simulink model "ConImpMulti2Robo_v1"  (R2015b)
settings: Solver=ode1  StartTime=0.0  StopTime=inf  FixedStep=0.005  RelTol=1e-3
undefined symbols (not defined in the file or in its folder): HIL
libraries: quarc_library x6, simulink x1
settings Model: SimulationMode=external  ExtModeTrigDuration=10000  Creator=rhuq  LastModifiedBy=anle
settings SolverCC: PositivePriorityOrder=on
settings DataIOCC: SaveFormat=Array  SignalLoggingSaveFormat=ModelDataLogs
settings OptimizationCC: ExpressionDepthLimit=2147483647  InitFltsAndDblsToZero=on
settings DebuggingCC: SaveWithParameterizedLinksMsg=none  UnderspecifiedInitializationDetection=Classic  MergeDetectMultiDrivingBlocksExec=none  SolverPrmCheckMsg=warning  ParameterPrecisionLossMsg=none  FcnCallInpInsideContextMsg=UseLocalSettings  StateNameClashWarn=warning
settings HardwareCC: ProdBitPerPointer=32  ProdLargestAtomicFloat=None  ProdIntDivRoundTo=Undefined  ProdEndianess=Unspecified  ProdWordSize=32  ProdHWDeviceType=32-bit Generic
settings SFSimCC: SimParseCustomCode=off
settings RTWCC: SystemTargetFile=quarc_linux_duovero.tlc  TemplateMakefile=quarc_linux_duovero_tmf  Description=QUARC Linux DuoVero Target
settings STFCustomTargetCC: TargetLibSuffix=.a  TargetPreCompLibLocation=C:\PROGRA~3\QUARC\lib\2015b\LINUX_~1\release  CombineOutputUpdateFcns=on  GRTInterface=off  SystemTargetFile=quarc_linux_duovero.tlc
settings GRTTargetCC: TargetLibSuffix=.a  TargetPreCompLibLocation=C:\PROGRA~3\QUARC\lib\2015b\LINUX_~1\release  ParMdlRefBuildCompliant=off  CompOptLevelCompliant=off  GeneratePreprocessorConditionals=Disable all  MatFileLogging=off  UseToolchainInfoCompliant=off  ExtMode=on  ExtModeMexFile=quarc_comm  ExtModeMexArgs='-w -d /tmp -uri %u' 'tcpip://192.168.2.49:17001'
settings ConfigComp: CovModelRefEnable=Off

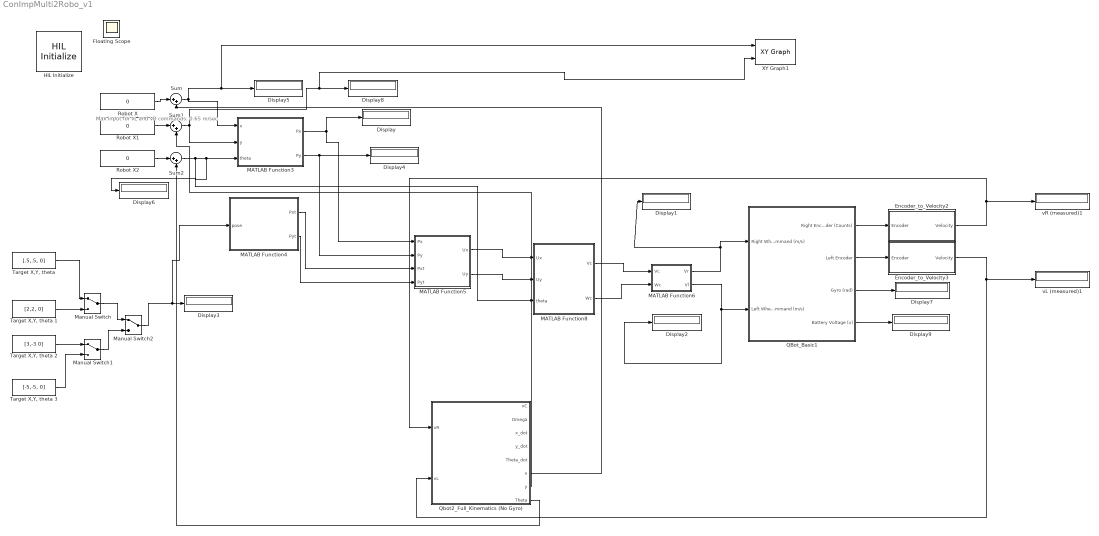
== system ConImpMulti2Robo_v1 ==
  note: Max input for vL and vR commands: 0.65 m/sec
  Display{,1..9} (10 alike) : Display
  Encoder_to_Velocity2 : Subsystem
  Encoder_to_Velocity3 : Subsystem
  HIL Initialize : quarc_library/Data Acquisition/Generic/Configuration/HIL Initialize  Priority=-99  object_name=HIL-1  board_type=qbot2  board_number=0  board_options=enc0_dir=0;enc0_filter=1;enc0_a=0;enc0_b=0;enc0_z=1;enc0_reload=0;enc1_dir=0;enc1_filter=1;enc1_a=0;enc1_b=0;enc1_z=1;enc1_reload=0;pwm0_immediate=0;pwm1_immediate=0;pwm2_immediate=0;pwm3_immediate=0;  exclusive=off  active=off  hardware_clocks=[]  clock_modes=[]  initial_clock_frequencies=[]  set_clock_params_at_start=off  set_clock_params_at_switch_in=off  set_clock_frequencies_at_start=off  set_clock_frequencies_at_switch_in=off  analog_input_channels=[0:9]  analog_input_maximums=[5 5 5 5 16.5 3.3 3.3 3.3 3.3]  analog_input_minimums=[0 0 0 0 0 0 0 0 0]  set_analog_input_params_at_start=off  set_analog_input_params_at_switch_in=off  analog_output_channels=[]  analog_output_maximums=[]  analog_output_minimums=[]  initial_analog_outputs=[]  final_analog_outputs=[]  watchdog_analog_outputs=[]  set_analog_output_params_at_start=off  set_analog_output_params_at_switch_in=off  set_analog_outputs_at_start=off  set_analog_outputs_at_switch_in=off  set_analog_outputs_at_terminate=off  set_analog_outputs_at_switch_out=off  set_analog_outputs_on_watchdog=off  digital_input_channels=[]  digital_output_channels=[]  digital_output_configuration=[]  initial_digital_outputs=[0]  final_digital_outputs=[0]  watchdog_digital_outputs=[0]  set_digital_output_params_at_start=off  set_digital_output_params_at_switch_in=off  set_digital_outputs_at_start=on  set_digital_outputs_at_switch_in=off  set_digital_outputs_at_terminate=on  set_digital_outputs_at_switch_out=off  set_digital_outputs_on_watchdog=on  encoder_channels=[0:3]  quadrature=[4]  encoder_filter_frequency=[]  initial_encoder_counts=[0]  set_encoder_params_at_start=on  set_encoder_params_at_switch_in=off  set_encoder_counts_at_start=on  set_encoder_counts_at_switch_in=off  pwm_channels=[0:3]  pwm_modes=[0 0 0 0]  pwm_frequency=[20e6/1024 20e6/1024 20e6/1024 20e6/1024]  pwm_configuration=[0]  pwm_alignment=[0]  pwm_polarity=[1]  pwm_leading_deadband=[0]  pwm_trailing_deadband=[0]  initial_pwm_outputs=[0]  final_pwm_outputs=[0]  watchdog_pwm_outputs=[0]  set_pwm_params_at_start=on  set_pwm_params_at_switch_in=off  set_pwm_outputs_at_start=on  set_pwm_outputs_at_switch_in=off  set_pwm_outputs_at_terminate=on  set_pwm_outputs_at_switch_out=off  set_pwm_outputs_on_watchdog=on  other_output_channels=[2000:2001]  initial_other_outputs=[0 0 7]  final_other_outputs=[0 0 1]  watchdog_other_outputs=[]  set_other_outputs_at_start=on  set_other_outputs_at_switch_in=off  set_other_outputs_at_terminate=on  set_other_outputs_at_switch_out=off  set_other_outputs_on_watchdog=off
  MATLAB Function3 : MATLAB Function  TreatAsAtomicUnit=on
  MATLAB Function4 : MATLAB Function  TreatAsAtomicUnit=on
  MATLAB Function5 : MATLAB Function  TreatAsAtomicUnit=on
  MATLAB Function6 : MATLAB Function  TreatAsAtomicUnit=on
  MATLAB Function8 : MATLAB Function  TreatAsAtomicUnit=on
  Manual Switch : ManualSwitch
  Manual Switch1 : ManualSwitch
  Manual Switch2 : ManualSwitch
  QBot_Basic1 : Subsystem
  Qbot2_Full_Kinematics (No Gyro) : Subsystem
  Robot X : Constant  Value=0
  Robot X1 : Constant  Value=0
  Robot X2 : Constant  Value=0
  Sum : Sum  Inputs=|++
  Sum1 : Sum  Inputs=|++
  Sum2 : Sum  Inputs=|++
  "Target X,Y, theta " : Constant  Value=[.5,.5, 0]
  "Target X,Y, theta 1" : Constant  Value=[2,2, 0]
  "Target X,Y, theta 2" : Constant  Value=[3,-3 0]
  "Target X,Y, theta 3" : Constant  Value=[-5,-5, 0]
  XY Graph1 : simulink/Sinks/XY Graph  xmin=-3  xmax=3  ymin=-3  ymax=3  st=-1
  vL (measured)1 : Display
  vR (measured)1 : Display
  Floating Scope : Scope
  wires:
  MATLAB Function4/1(Pxt) -> MATLAB Function5/3(Pxt)
  MATLAB Function4/2(Pyt) -> MATLAB Function5/4(Pyt)
  MATLAB Function3/2(Py) -> MATLAB Function5/2(Py), Display4/1
  MATLAB Function3/1(Px) -> MATLAB Function5/1(Px), Display/1
  Sum2/1 -> MATLAB Function8/3(theta), Display6/1, MATLAB Function3/3(theta)
  Robot X2/1 -> Sum2/1
  Robot X/1 -> Sum/1
  Robot X1/1 -> Sum1/1
  Manual Switch2/1 -> MATLAB Function4/1(pose), Display3/1
  "Target X,Y, theta "/1 -> Manual Switch/1
  "Target X,Y, theta 1"/1 -> Manual Switch/2
  Manual Switch/1 -> Manual Switch2/1
  Manual Switch1/1 -> Manual Switch2/2
  "Target X,Y, theta 2"/1 -> Manual Switch1/1
  "Target X,Y, theta 3"/1 -> Manual Switch1/2
  MATLAB Function5/1(Ux) -> MATLAB Function8/1(Ux)
  MATLAB Function5/2(Uy) -> MATLAB Function8/2(Uy)
  MATLAB Function8/1(Vc) -> MATLAB Function6/1(Vc)
  MATLAB Function8/2(Wc) -> MATLAB Function6/2(Wc)
  MATLAB Function6/1(Vr) -> Display1/1, QBot_Basic1/1(Right Wheel Command (m/s))
  MATLAB Function6/2(Vl) -> Display2/1, QBot_Basic1/2(Left Wheel Command (m/s))
  QBot_Basic1/1(Right Encoder (Counts)) -> Encoder_to_Velocity2/1(Encoder)
  QBot_Basic1/2(Left Encoder) -> Encoder_to_Velocity3/1(Encoder)
  QBot_Basic1/3(Gyro (rad)) -> Display7/1
  QBot_Basic1/4(Battery Voltage (v)) -> Display9/1
  Encoder_to_Velocity2/1(Velocity) -> Qbot2_Full_Kinematics (No Gyro)/1(vR), vR (measured)1/1
  Encoder_to_Velocity3/1(Velocity) -> Qbot2_Full_Kinematics (No Gyro)/2(vL), vL (measured)1/1
  Sum1/1 -> MATLAB Function3/2(y), XY Graph1/2, Display8/1
  Sum/1 -> MATLAB Function3/1(x), XY Graph1/1, Display5/1
  Qbot2_Full_Kinematics (No Gyro)/6(x) -> Sum/2
  Qbot2_Full_Kinematics (No Gyro)/7(y) -> Sum1/2
  Qbot2_Full_Kinematics (No Gyro)/8(Theta) -> Sum2/2

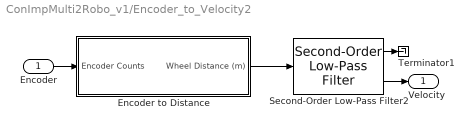
== system ConImpMulti2Robo_v1/Encoder_to_Velocity2 ==
  Encoder : Inport
  Encoder to Distance : Subsystem
  Second-Order Low-Pass Filter2 : quarc_library/Continuous/Second-Order Low-Pass Filter  params_source=Internal (dialog parameters)  input_width=10  input_zeta=1  input_init=0
  Terminator1 : Terminator
  Velocity : Outport
  wires:
  Second-Order Low-Pass Filter2/2 -> Velocity/1
  Encoder/1 -> Encoder to Distance/1(Encoder Counts)
  Encoder to Distance/1(Wheel Distance (m)) -> Second-Order Low-Pass Filter2/1
  Second-Order Low-Pass Filter2/1 -> Terminator1/1

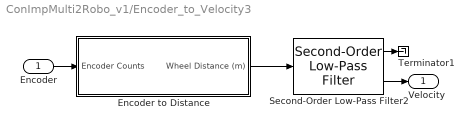
== system ConImpMulti2Robo_v1/Encoder_to_Velocity3 ==
  Encoder : Inport
  Encoder to Distance : Subsystem
  Second-Order Low-Pass Filter2 : quarc_library/Continuous/Second-Order Low-Pass Filter  params_source=Internal (dialog parameters)  input_width=10  input_zeta=1  input_init=0
  Terminator1 : Terminator
  Velocity : Outport
  wires:
  Second-Order Low-Pass Filter2/2 -> Velocity/1
  Encoder/1 -> Encoder to Distance/1(Encoder Counts)
  Encoder to Distance/1(Wheel Distance (m)) -> Second-Order Low-Pass Filter2/1
  Second-Order Low-Pass Filter2/1 -> Terminator1/1

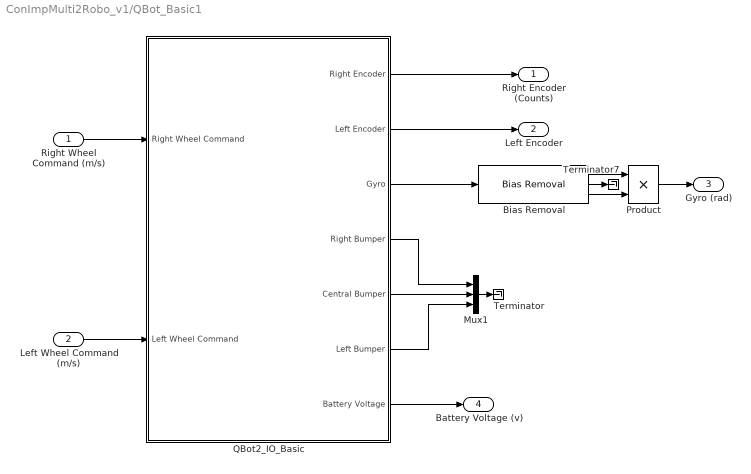
== system ConImpMulti2Robo_v1/QBot_Basic1 ==
  Right Wheel Command (m/s) : Inport
  Left Wheel Command (m/s) : Inport  Port=2
  Bias Removal : quarc_library/Discrete/Bias Removal  start_time=3  end_time=4  switch_id=0  sample_time=qc_get_step_size
  Mux1 : Mux  Inputs=3
  Product : Product  RndMeth=Zero
  QBot2_IO_Basic : Subsystem
  Terminator : Terminator
  Terminator7 : Terminator
  Right Encoder (Counts) : Outport
  Left Encoder : Outport  Port=2
  Gyro (rad) : Outport  Port=3
  Battery Voltage (v) : Outport  Port=4
  wires:
  Mux1/1 -> Terminator/1
  QBot2_IO_Basic/3(Gyro) -> Bias Removal/1
  Product/1 -> Gyro (rad)/1
  Bias Removal/3 -> Product/2
  Bias Removal/1 -> Product/1
  Bias Removal/2 -> Terminator7/1
  QBot2_IO_Basic/7(Battery Voltage) -> Battery Voltage (v)/1
  QBot2_IO_Basic/2(Left Encoder) -> Left Encoder/1
  QBot2_IO_Basic/1(Right Encoder) -> Right Encoder (Counts)/1
  Left Wheel Command (m/s)/1 -> QBot2_IO_Basic/2(Left Wheel Command)
  Right Wheel Command (m/s)/1 -> QBot2_IO_Basic/1(Right Wheel Command)
  QBot2_IO_Basic/6(Left Bumper) -> Mux1/3
  QBot2_IO_Basic/5(Central Bumper) -> Mux1/2
  QBot2_IO_Basic/4(Right Bumper) -> Mux1/1

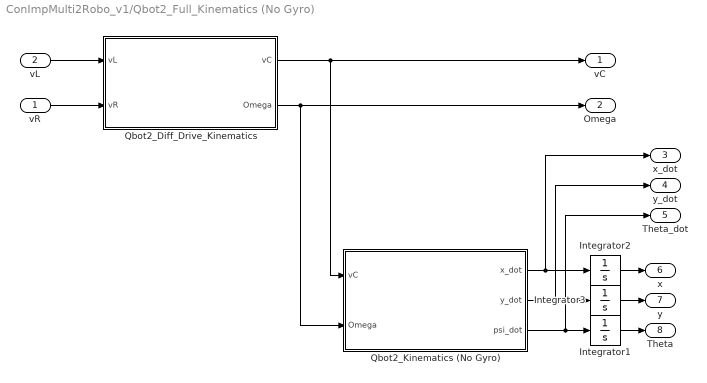
== system ConImpMulti2Robo_v1/Qbot2_Full_Kinematics (No Gyro) ==
  vR : Inport
  vL : Inport  Port=2
  Integrator1 : Integrator
  Integrator2 : Integrator
  Integrator3 : Integrator
  Qbot2_Diff_Drive_Kinematics : Subsystem
  Qbot2_Kinematics (No Gyro) : Subsystem
  vC : Outport
  Omega : Outport  Port=2
  x_dot : Outport  Port=3
  y_dot : Outport  Port=4
  Theta_dot : Outport  Port=5
  x : Outport  Port=6
  y : Outport  Port=7
  Theta : Outport  Port=8
  wires:
  Qbot2_Diff_Drive_Kinematics/2(Omega) -> Omega/1, Qbot2_Kinematics (No Gyro)/2(Omega)
  Integrator3/1 -> y/1
  Integrator2/1 -> x/1
  vR/1 -> Qbot2_Diff_Drive_Kinematics/2(vR)
  vL/1 -> Qbot2_Diff_Drive_Kinematics/1(vL)
  Qbot2_Diff_Drive_Kinematics/1(vC) -> vC/1, Qbot2_Kinematics (No Gyro)/1(vC)
  Qbot2_Kinematics (No Gyro)/2(y_dot) -> Integrator3/1, y_dot/1
  Qbot2_Kinematics (No Gyro)/1(x_dot) -> Integrator2/1, x_dot/1
  Qbot2_Kinematics (No Gyro)/3(psi_dot) -> Integrator1/1, Theta_dot/1
  Integrator1/1 -> Theta/1

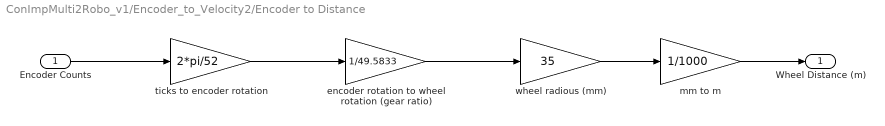
== system ConImpMulti2Robo_v1/Encoder_to_Velocity2/Encoder to Distance ==
  Encoder Counts : Inport
  " encoder rotation to wheel rotation (gear ratio)" : Gain  Gain=1/49.5833
  mm to m : Gain  Gain=1/1000
  ticks to encoder rotation : Gain  Gain=2*pi/52
  wheel radious (mm) : Gain  Gain=35
  Wheel Distance (m) : Outport
  wires:
  mm to m/1 -> Wheel Distance (m)/1
  wheel radious (mm)/1 -> mm to m/1
  " encoder rotation to wheel rotation (gear ratio)"/1 -> wheel radious (mm)/1
  ticks to encoder rotation/1 -> " encoder rotation to wheel rotation (gear ratio)"/1
  Encoder Counts/1 -> ticks to encoder rotation/1

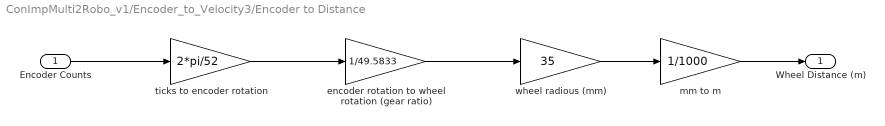
== system ConImpMulti2Robo_v1/Encoder_to_Velocity3/Encoder to Distance ==
  Encoder Counts : Inport
  " encoder rotation to wheel rotation (gear ratio)" : Gain  Gain=1/49.5833
  mm to m : Gain  Gain=1/1000
  ticks to encoder rotation : Gain  Gain=2*pi/52
  wheel radious (mm) : Gain  Gain=35
  Wheel Distance (m) : Outport
  wires:
  mm to m/1 -> Wheel Distance (m)/1
  wheel radious (mm)/1 -> mm to m/1
  " encoder rotation to wheel rotation (gear ratio)"/1 -> wheel radious (mm)/1
  ticks to encoder rotation/1 -> " encoder rotation to wheel rotation (gear ratio)"/1
  Encoder Counts/1 -> ticks to encoder rotation/1

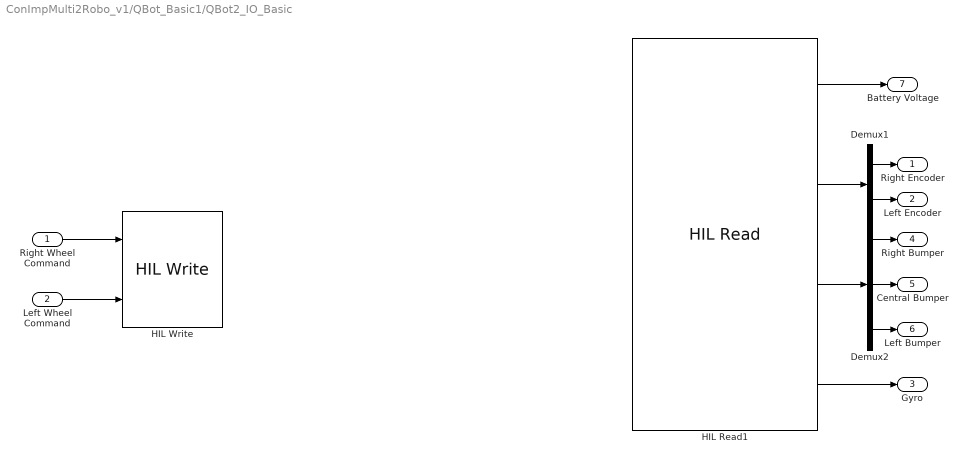
== system ConImpMulti2Robo_v1/QBot_Basic1/QBot2_IO_Basic ==
  Right Wheel Command : Inport
  Left Wheel Command : Inport  Port=2
  Demux1 : Demux  Outputs=2
  Demux2 : Demux  Outputs=3
  HIL Read1 : quarc_library/Data Acquisition/Generic/Immediate I//O/HIL Read  object_name=HIL-1  analog_channels=[4]  encoder_channels=[2 3]  digital_channels=[8 9 10]  other_channels=[1002]  sample_time=qc_get_step_size  active=on  vector_output=on  data_type_mode=Inherit via back propagation  encoder_data_type=double  digital_data_type=boolean
  HIL Write : quarc_library/Data Acquisition/Generic/Immediate I//O/HIL Write  object_name=HIL-1  analog_channels=[]  pwm_channels=[]  digital_channels=[]  other_channels=[2000:2001]  sample_time=-1  active=on  vector_input=off
  Right Encoder : Outport
  Left Encoder : Outport  Port=2
  Gyro : Outport  Port=3
  Right Bumper : Outport  Port=4
  Central Bumper : Outport  Port=5
  Left Bumper : Outport  Port=6
  Battery Voltage : Outport  Port=7
  wires:
  Demux2/3 -> Left Bumper/1
  Demux2/2 -> Central Bumper/1
  Demux2/1 -> Right Bumper/1
  HIL Read1/2 -> Demux1/1
  Left Wheel Command/1 -> HIL Write/2
  Right Wheel Command/1 -> HIL Write/1
  Demux1/2 -> Left Encoder/1
  Demux1/1 -> Right Encoder/1
  HIL Read1/4 -> Gyro/1
  HIL Read1/3 -> Demux2/1
  HIL Read1/1 -> Battery Voltage/1

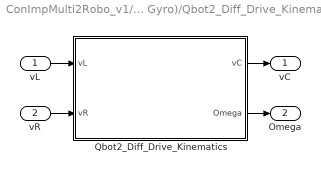
== system ConImpMulti2Robo_v1/Qbot2_Full_Kinematics (No Gyro)/Qbot2_Diff_Drive_Kinematics ==
  vL : Inport
  vR : Inport  Port=2
  Qbot2_Diff_Drive_Kinematics : MATLAB Function  TreatAsAtomicUnit=on
  vC : Outport
  Omega : Outport  Port=2
  wires:
  Qbot2_Diff_Drive_Kinematics/2(Omega) -> Omega/1
  vR/1 -> Qbot2_Diff_Drive_Kinematics/2(vR)
  Qbot2_Diff_Drive_Kinematics/1(vC) -> vC/1
  vL/1 -> Qbot2_Diff_Drive_Kinematics/1(vL)

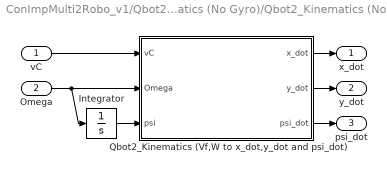
== system ConImpMulti2Robo_v1/Qbot2_Full_Kinematics (No Gyro)/Qbot2_Kinematics (No Gyro) ==
  vC : Inport
  Omega : Inport  Port=2
  Integrator : Integrator
  Qbot2_Kinematics (Vf,W to x_dot,y_dot and psi_dot) : MATLAB Function  TreatAsAtomicUnit=on
  x_dot : Outport
  y_dot : Outport  Port=2
  psi_dot : Outport  Port=3
  wires:
  Qbot2_Kinematics (Vf,W to x_dot,y_dot and psi_dot)/2(y_dot) -> y_dot/1
  Omega/1 -> Qbot2_Kinematics (Vf,W to x_dot,y_dot and psi_dot)/2(Omega), Integrator/1
  Qbot2_Kinematics (Vf,W to x_dot,y_dot and psi_dot)/1(x_dot) -> x_dot/1
  vC/1 -> Qbot2_Kinematics (Vf,W to x_dot,y_dot and psi_dot)/1(vC)
  Integrator/1 -> Qbot2_Kinematics (Vf,W to x_dot,y_dot and psi_dot)/3(psi)
  Qbot2_Kinematics (Vf,W to x_dot,y_dot and psi_dot)/3(psi_dot) -> psi_dot/1

== matlab function ConImpMulti2Robo_v1/Qbot2_Full_Kinematics (No Gyro)/Qbot2_Diff_Drive_Kinematics/Qbot2_Diff_Drive_Kinematics ==
  data: vL input; vC output; vR input; Omega output
function [vC,Omega] = fcn(vL,vR)
%#codegen

d= 0.235;

vC=0.5*(vL+vR);
Omega=(1/d)*(vR-vL);

== matlab function ConImpMulti2Robo_v1/Qbot2_Full_Kinematics (No Gyro)/Qbot2_Kinematics (No Gyro)/Qbot2_Kinematics (Vf,W to x_dot,y_dot and psi_dot) ==
  data: vC input; x_dot output; Omega input; y_dot output; psi input; psi_dot output
function [x_dot,y_dot,psi_dot] = fcn(vC,Omega,psi)
%#codegen


x_dot=cos(psi)*vC;
y_dot=sin(psi)*vC;
psi_dot= Omega;

== matlab function ConImpMulti2Robo_v1/MATLAB Function3 ==
  data: x input; Px output; Py output; y input; theta input
function [Px,Py] = PxPy_convert(x, y, theta)

l=.0235; %#length between the two wheels in meters
%R=.0175; %#R or signed distance from ICC (Instanteous center of curvature) in meters
Px= x+l*cos(theta)
Py = y+l*sin(theta)

%#codegen

== matlab function ConImpMulti2Robo_v1/MATLAB Function4 ==
  data: pose input; Pxt output; Pyt output
function [Pxt,Pyt] = PxtPyt_convert(pose)
x=pose(1);
y=pose(2);
theta=pose(2);
l=.0235; %#length between the two wheels in meters
%R=.0175; %#R or signed distance from ICC (Instanteous center of curvature) in meters
Pxt= x+l*cos(theta)
Pyt = y+l*sin(theta)

%#codegen

== matlab function ConImpMulti2Robo_v1/MATLAB Function6 ==
  data: Vc input; Vr output; Wc input; Vl output
function [Vr,Vl] = VcWc2VrVl(Vc,Wc)
%#codegen

l=.0235;
Vr = Vc+(1/2)*(l*2)*Wc;
Vl = Vc-(1/2)*(l*2)*Wc;

== matlab function ConImpMulti2Robo_v1/MATLAB Function5 ==
  data: Px input; Ux output; Py input; Pxt input; Pyt input; Uy output
function [Ux, Uy] = UxUy(Px,Py,Pxt,Pyt)
%#codegen
%rho_star=.5;
%omega_star=.5;
 
krho = .75;
kphi = 1;
w_d=.05;
 
U = [0 0];
rho_size = .5;
phi_size = 1;
[phi, rho] = cart2pol(Px,Py);
[phi_d, rho_d] = cart2pol(Pxt,Pyt);
 
[phi_dif, rho_dif] = cart2pol((Px-Pxt),(Py-Pyt));
 
PxD = Px - Pxt; 
PyD = Py - Pyt;
 
 
 
J_i=[PxD/(sqrt(PxD^2+PyD^2)) PyD/(sqrt(PxD^2+PyD^2)); -PyD/(PxD^2+PyD^2) PxD/(PxD^2+PyD^2)];
 
 
 
 
%J_i=[(Px-Pxt)/phi_dif (Py-Pyt)/phi_dif;...
%    -(Py-Pyt)/((1+((Py-Pyt)/(PD))^2)*(Px-Pxt)^2)  1/((1+((Py-Pyt)/(PD))^2)*(Px-Pxt))];
 
 
 
%J_i=[ (Px-Pxt)/phi (Py-Pyt)/phi_dif;    -(Py-Pyt)/(phi_dif)^2  (Px-Pxt)/(phi_dif)^2 ];
 
rhoi_dot = krho*(rho_size-rho_dif)
%phii_d= phi/2
%phii_d = phi_d - phii_d
phii_dot = w_d; %+ kphi*((phi_size-phi)/2);
V_i= [rhoi_dot; phii_dot];
Rt = [ 1 0; 0 1];
 
 
U = Rt*(J_i'*V_i);
U = inv(J_i)*V_i; 
Ux = U(1);
Uy = U(2);

== matlab function ConImpMulti2Robo_v1/MATLAB Function8 ==
  data: Ux input; Vc output; Uy input; Wc output; theta input
function [Vc,Wc] = UxUy2VcWc(Ux,Uy, theta)

l=.0235; %#length between the two wheels in meters
kin_inv = inv([cos(theta) -l*sin(theta) ; sin(theta) l*cos(theta)]);
P =  kin_inv*[Ux;Uy];
Vc=P(1);
Wc=P(2);
